simulink library "GFL_Lib"  (R2021a)
settings: Solver=VariableStepAuto  StartTime=0.0  StopTime=10.0  RelTol=1e-3
values from neighbouring files (symbols this model uses):
  Ki_i = Rc_eq*wn_i    [Init_GFL.m]
  Kp_i = Lc_eq/wb*wn_i    [Init_GFL.m]
  Lc_eq = Lc_pu + dLc_pu    [Init_VI_mmc.m]
  Lc_pu = Lt_pu+Larm_pu/2    [Init_VI_mmc.m]
  Lf_pu = Lc_eq    [Init_GFL.m]
  Va0 = sqrt(2)*Vb1*Vvsc0*sin(Theta_vsc0*pi/180)    [Init_LF_LCL_old.m]
  Vb0 = sqrt(2)*Vb1*Vvsc0*sin(Theta_vsc0*pi/180-2*pi/3)    [Init_LF_LCL_old.m]
  Vc0 = sqrt(2)*Vb1*Vvsc0*sin(Theta_vsc0*pi/180+2*pi/3)    [Init_LF_LCL_old.m]
  Vm0_d = Vvsc0 * cos(Theta_vsc0*pi/180-Theta_m0*pi/180)    [Init_LF_LCL_old.m]
  Vm0_q = Vvsc0 * sin(Theta_vsc0*pi/180-Theta_m0*pi/180)    [Init_LF_LCL_old.m]
  Vvsc0 = abs(Vm)    [Init_LF_LCL_old.m]
undefined symbols (not defined in the file or in its folder): Carm, Diff_CC_ki, Diff_CC_kp, fb, Ib2, Idcb, Ki_Wdiff_pu, Ki_Wtot_pu, Kp_Rvi_pu, Kp_Wdiff_pu, Kp_Wtot_pu, Lb, Sb, Solver_Time_Step, Time_Step, Vb1, Vb2, Vdcb, Vm0, VSC01_id0, wb, Zb
libraries: Control_Lib x57, spsVoltageMeasurementLib x17, spsSeriesRLCBranchLib x14, spsThreePhaseSourceLib x12, spsThreePhaseBreakerLib x10, spsThreePhaseVIMeasurementLib x9, spsThreePhaseTransformerTwoWindingsLib x7, spsCurrentMeasurementLib x7, powerlib x7, spsControlledCurrentSourceLib x6, spsControlledVoltageSourceLib x6, slpidlib x6
(part 5 of 6)

== system GFL_Lib/Mean Model 2-Level L-filter_old/Control loops/LPF3 ==
  In1 : Inport
  Add : Sum  Inputs=+-
  Gain : Gain  Gain=2*pi*50
  Integrator : Integrator  InitialCondition=V0
  Out1 : Outport
  wires:
  In1/1 -> Add/1
  Integrator/1 -> Add/2, Out1/1
  Gain/1 -> Integrator/1
  Add/1 -> Gain/1

== system GFL_Lib/Mean Model 2-Level L-filter_old/Control loops/RMS derivation ==
  dq : Inport
  Demux : Demux  Outputs=2
  Sqrt : Sqrt  SaturateOnIntegerOverflow=on
  Square : Math  Operator=square  SaturateOnIntegerOverflow=on
  Square1 : Math  Operator=square  SaturateOnIntegerOverflow=on
  Sum : Sum
  rms : Outport
  wires:
  dq/1 -> Demux/1
  Demux/2 -> Square1/1
  Square/1 -> Sum/1
  Demux/1 -> Square/1
  Sqrt/1 -> rms/1
  Sum/1 -> Sqrt/1
  Square1/1 -> Sum/2

== system GFL_Lib/Mean Model 2-Level L-filter_old/Control loops/norm1 ==
  In1 : Inport
  Add : Sum
  Demux : Demux  Outputs=2
  Sqrt : Sqrt  SaturateOnIntegerOverflow=on
  Square : Math  Operator=square  SaturateOnIntegerOverflow=on
  Square1 : Math  Operator=square  SaturateOnIntegerOverflow=on
  Out1 : Outport
  wires:
  In1/1 -> Demux/1
  Square1/1 -> Add/2
  Square/1 -> Add/1
  Demux/1 -> Square/1
  Demux/2 -> Square1/1
  Add/1 -> Sqrt/1
  Sqrt/1 -> Out1/1

== system GFL_Lib/Mean Model 2-Level L-filter_old/Control loops/norm2 ==
  In1 : Inport
  Add : Sum
  Demux : Demux  Outputs=2
  Sqrt : Sqrt  SaturateOnIntegerOverflow=on
  Square : Math  Operator=square  SaturateOnIntegerOverflow=on
  Square1 : Math  Operator=square  SaturateOnIntegerOverflow=on
  Out1 : Outport
  wires:
  In1/1 -> Demux/1
  Square1/1 -> Add/2
  Square/1 -> Add/1
  Demux/1 -> Square/1
  Demux/2 -> Square1/1
  Add/1 -> Sqrt/1
  Sqrt/1 -> Out1/1

== system GFL_Lib/Mean Model 2-Level L-filter_sav/Control loops/ pu P//Q computation ==
  v_abc_pu : Inport  PortDimensions=3
  i_abc_pu : Inport  Port=2  PortDimensions=3
  Demux : Demux  Outputs=3
      settings: DisplayOption=none
  Mux : Mux  Inputs=3
  Product1 : Product  InputSameDT=on  SaturateOnIntegerOverflow=on  OutDataTypeStr=Inherit: Same as first input
  Product3 : Product  InputSameDT=on  SaturateOnIntegerOverflow=on  OutDataTypeStr=Inherit: Same as first input
  Sum : Sum  Inputs=+-  InputSameDT=on  SaturateOnIntegerOverflow=on  OutDataTypeStr=Inherit: Same as first input
  Sum1 : Sum  Inputs=1  InputSameDT=on  SaturateOnIntegerOverflow=on  OutDataTypeStr=Inherit: Same as first input
  Sum4 : Sum  Inputs=1  InputSameDT=on  SaturateOnIntegerOverflow=on  OutDataTypeStr=Inherit: Same as first input
  Sum5 : Sum  Inputs=+-  InputSameDT=on  SaturateOnIntegerOverflow=on  OutDataTypeStr=Inherit: Same as first input
  Sum6 : Sum  Inputs=+-  InputSameDT=on  SaturateOnIntegerOverflow=on  OutDataTypeStr=Inherit: Same as first input
  pu->V : Gain  Gain=1/sqrt(3)  SaturateOnIntegerOverflow=on  OutDataTypeStr=Inherit: Same as input  ParamDataTypeStr=Inherit: Same as input
  pu->V1 : Gain  Gain=1/3  SaturateOnIntegerOverflow=on  OutDataTypeStr=Inherit: Same as input  ParamDataTypeStr=Inherit: Same as input
  pu->V2 : Gain  Gain=1/3  SaturateOnIntegerOverflow=on  OutDataTypeStr=Inherit: Same as input  ParamDataTypeStr=Inherit: Same as input
  P : Outport  VectorParamsAs1DForOutWhenUnconnected=off
  Q : Outport  Port=2  VectorParamsAs1DForOutWhenUnconnected=off
  wires:
  pu->V2/1 -> Q/1
  pu->V1/1 -> P/1
  Sum1/1 -> pu->V/1
  Product3/1 -> Sum1/1
  Product1/1 -> Sum4/1
  v_abc_pu/1 -> Product1/1, Demux/1
  i_abc_pu/1 -> Product1/2, Product3/2
  Sum4/1 -> pu->V1/1
  Demux/1 -> Sum/1, Sum6/2
  Demux/2 -> Sum/2, Sum5/1
  Demux/3 -> Sum5/2, Sum6/1
  Sum/1 -> Mux/3
  Sum5/1 -> Mux/1
  Sum6/1 -> Mux/2
  Mux/1 -> Product3/1
  pu->V/1 -> pu->V2/1  "Q"

== system GFL_Lib/Mean Model 2-Level L-filter_sav/Control loops/Inner Current Control ==
  ig_dq_ref : Inport
  ig_dq : Inport  Port=2
  theta_PLL : Inport  Port=3
  w_PLL : Inport  Port=4
  vg_dq : Inport  Port=5
  Control Delay compensation : Constant  Value=wb*Solver_Time_Step
  Current PI control : Subsystem
  Mux : Mux  Inputs=2
  Sum : Sum  Inputs=|++
  Trigonometric Function : Trigonometry
  Trigonometric Function1 : Trigonometry  Operator=cos
  vm_dq : Outport  VectorParamsAs1DForOutWhenUnconnected=off
  CosSinTheta_delay : Outport  Port=2  VectorParamsAs1DForOutWhenUnconnected=off
  wires:
  ig_dq/1 -> Current PI control/1(Is_dq)  "Is_dq"
  Current PI control/1(vm_dq_ref) -> vm_dq/1  "vm_dq"
  ig_dq_ref/1 -> Current PI control/3(Is_dq_ref)
  vg_dq/1 -> Current PI control/2(Eg_dqfr)  "Eg_dq"
  w_PLL/1 -> Current PI control/4(w)  "w"
  Control Delay compensation/1 -> Sum/2
  Trigonometric Function/1 -> Mux/2
  Sum/1 -> Trigonometric Function/1, Trigonometric Function1/1
  theta_PLL/1 -> Sum/1  "Theta"
  Trigonometric Function1/1 -> Mux/1
  Mux/1 -> CosSinTheta_delay/1

== system GFL_Lib/Mean Model 2-Level LCL-filter [under construction]/Control loops/ pu P//Q computation ==
  v_abc_pu : Inport  PortDimensions=3
  i_abc_pu : Inport  Port=2  PortDimensions=3
  Demux : Demux  Outputs=3
      settings: DisplayOption=none
  Mux : Mux  Inputs=3
  Product1 : Product  InputSameDT=on  SaturateOnIntegerOverflow=on  OutDataTypeStr=Inherit: Same as first input
  Product3 : Product  InputSameDT=on  SaturateOnIntegerOverflow=on  OutDataTypeStr=Inherit: Same as first input
  Sum : Sum  Inputs=+-  InputSameDT=on  SaturateOnIntegerOverflow=on  OutDataTypeStr=Inherit: Same as first input
  Sum1 : Sum  Inputs=1  InputSameDT=on  SaturateOnIntegerOverflow=on  OutDataTypeStr=Inherit: Same as first input
  Sum4 : Sum  Inputs=1  InputSameDT=on  SaturateOnIntegerOverflow=on  OutDataTypeStr=Inherit: Same as first input
  Sum5 : Sum  Inputs=+-  InputSameDT=on  SaturateOnIntegerOverflow=on  OutDataTypeStr=Inherit: Same as first input
  Sum6 : Sum  Inputs=+-  InputSameDT=on  SaturateOnIntegerOverflow=on  OutDataTypeStr=Inherit: Same as first input
  pu->V : Gain  Gain=1/sqrt(3)  SaturateOnIntegerOverflow=on  OutDataTypeStr=Inherit: Same as input  ParamDataTypeStr=Inherit: Same as input
  pu->V1 : Gain  Gain=1/3  SaturateOnIntegerOverflow=on  OutDataTypeStr=Inherit: Same as input  ParamDataTypeStr=Inherit: Same as input
  pu->V2 : Gain  Gain=1/3  SaturateOnIntegerOverflow=on  OutDataTypeStr=Inherit: Same as input  ParamDataTypeStr=Inherit: Same as input
  P : Outport  VectorParamsAs1DForOutWhenUnconnected=off
  Q : Outport  Port=2  VectorParamsAs1DForOutWhenUnconnected=off
  wires:
  pu->V2/1 -> Q/1
  pu->V1/1 -> P/1
  Sum1/1 -> pu->V/1
  Product3/1 -> Sum1/1
  Product1/1 -> Sum4/1
  v_abc_pu/1 -> Product1/1, Demux/1
  i_abc_pu/1 -> Product1/2, Product3/2
  Sum4/1 -> pu->V1/1
  Demux/1 -> Sum/1, Sum6/2
  Demux/2 -> Sum/2, Sum5/1
  Demux/3 -> Sum5/2, Sum6/1
  Sum/1 -> Mux/3
  Sum5/1 -> Mux/1
  Sum6/1 -> Mux/2
  Mux/1 -> Product3/1
  pu->V/1 -> pu->V2/1  "Q"

== system GFL_Lib/Mean Model 2-Level LCL-filter [under construction]/Control loops/Inner Current Control ==
  ig_dq_ref : Inport
  ig_dq : Inport  Port=2
  theta_PLL : Inport  Port=3
  w_PLL : Inport  Port=4
  vg_dq : Inport  Port=5
  Current PI control : Subsystem
  vm_dq : Outport  VectorParamsAs1DForOutWhenUnconnected=off
  theta : Outport  Port=2  VectorParamsAs1DForOutWhenUnconnected=off
  wires:
  ig_dq/1 -> Current PI control/1(Is_dq)  "Is_dq"
  theta_PLL/1 -> theta/1  "Theta"
  Current PI control/1(vm_dq_ref) -> vm_dq/1  "vm_dq"
  ig_dq_ref/1 -> Current PI control/3(Is_dq_ref)
  vg_dq/1 -> Current PI control/2(Eg_dqfr)  "Eg_dq"
  w_PLL/1 -> Current PI control/4(w)  "w"

== system GFL_Lib/GFL IDEAL VSC/Control loops/Inner Current Control/LPF1 ==
  In1 : Inport
  Add : Sum  Inputs=+-
  Gain : Gain  Gain=w_ff
  Integrator : Integrator  InitialConditionSource=external  InitialCondition=V0*cos(Theta0*pi/180)
  Out1 : Outport
  wires:
  Add/1 -> Gain/1
  Gain/1 -> Integrator/1
  Integrator/1 -> Out1/1, Add/2
  In1/1 -> Integrator/2, Add/1

== system GFL_Lib/GFL IDEAL VSC/Control loops/Inner Current Control/LPF2 ==
  In1 : Inport
  Add : Sum  Inputs=+-
  Gain : Gain  Gain=w_ff
  Integrator : Integrator  InitialCondition=V0*sin(Theta0*pi/180)
  Out1 : Outport
  wires:
  Add/1 -> Gain/1
  Gain/1 -> Integrator/1
  Integrator/1 -> Out1/1, Add/2
  In1/1 -> Add/1

== system GFL_Lib/GFL MMC/Control loops/Inner Current Control/LPF1 ==
  In1 : Inport
  Add : Sum  Inputs=+-
  Gain : Gain  Gain=w_ff
  Integrator : Integrator  InitialConditionSource=external  InitialCondition=V0*cos(Theta0*pi/180)
  Out1 : Outport
  wires:
  Add/1 -> Gain/1
  Gain/1 -> Integrator/1
  Integrator/1 -> Out1/1, Add/2
  In1/1 -> Integrator/2, Add/1

== system GFL_Lib/GFL MMC/Control loops/Inner Current Control/LPF2 ==
  In1 : Inport
  Add : Sum  Inputs=+-
  Gain : Gain  Gain=w_ff
  Integrator : Integrator  InitialCondition=V0*sin(Theta0*pi/180)
  Out1 : Outport
  wires:
  Add/1 -> Gain/1
  Gain/1 -> Integrator/1
  Integrator/1 -> Out1/1, Add/2
  In1/1 -> Add/1

== system GFL_Lib/GFM_VC MMC/Bridge_Model/MMC Average Model/Arm_la ==
  m : Inport
  Controlled Current Source : spsControlledCurrentSourceLib/Controlled Current Source  Initialize=on  Source_Type=DC  Amplitude=0  Phase=0  Frequency=0  Measurements=None
  Controlled Voltage Source2 : spsControlledVoltageSourceLib/Controlled Voltage Source  Initialize=on  Source_Type=DC  Amplitude=Vdc/2  Phase=180  Frequency=0  Measurements=None
  Current Measurement7 : spsCurrentMeasurementLib/Current Measurement  PhasorSimulation=off  OutputType=Complex  PSBequivalent=0
  Memory1 : Memory  InitialCondition=Vdc/2
  Memory2 : Memory
  Product : Product  RndMeth=Zero
  Product1 : Product  RndMeth=Zero
  Series RLC Branch : spsSeriesRLCBranchLib/Series RLC Branch  LConnTagsString=__new0  RConnTagsString=__new0  BranchType=C  Resistance=1  Inductance=1e-3  SetiL0=off  InitialCurrent=0  Capacitance=C_arm  Setx0=on  InitialVoltage=Vdc  Measurements=None
  Voltage Measurement : spsVoltageMeasurementLib/Voltage Measurement  PhasorSimulation=off  OutputType=Complex  PSBequivalent=0
  Voltage Measurement1 : spsVoltageMeasurementLib/Voltage Measurement  PhasorSimulation=off  OutputType=Complex  PSBequivalent=0
  V+ : PMIOPort  Side=Left
  V- : PMIOPort  Port=2  Side=Left
  vctot : Outport
  i_arm : Outport  Port=2
  v_arm : Outport  Port=3
  wires:
  Memory1/1 -> Controlled Voltage Source2/1
  Memory2/1 -> Controlled Current Source/1
  Product/1 -> Memory1/1
  Voltage Measurement/1 -> v_arm/1
  Product1/1 -> Memory2/1
  m/1 -> [m], Product1/1
  Current Measurement7/1 -> i_arm/1, Product1/2
  [m] -> Product/2
  Voltage Measurement1/1 -> Product/1, vctot/1
  connections:
  Current Measurement7/RConn1 -- Controlled Voltage Source2/RConn1
  Current Measurement7/LConn1 -- Voltage Measurement/LConn1 -- V+/RConn1
  Controlled Current Source/LConn1 -- Series RLC Branch/RConn1 -- Voltage Measurement1/LConn2 -- V-/RConn1 -- Voltage Measurement/LConn2 -- Controlled Voltage Source2/LConn1
  Controlled Current Source/RConn1 -- Series RLC Branch/LConn1 -- Voltage Measurement1/LConn1

== system GFL_Lib/GFM_VC MMC/Bridge_Model/MMC Average Model/Arm_lb ==
  m : Inport
  Controlled Current Source : spsControlledCurrentSourceLib/Controlled Current Source  Initialize=on  Source_Type=DC  Amplitude=0  Phase=0  Frequency=0  Measurements=None
  Controlled Voltage Source2 : spsControlledVoltageSourceLib/Controlled Voltage Source  Initialize=on  Source_Type=DC  Amplitude=Vdc/2  Phase=180  Frequency=0  Measurements=None
  Current Measurement7 : spsCurrentMeasurementLib/Current Measurement  PhasorSimulation=off  OutputType=Complex  PSBequivalent=0
  Memory1 : Memory  InitialCondition=Vdc/2
  Memory2 : Memory
  Product : Product  RndMeth=Zero
  Product1 : Product  RndMeth=Zero
  Series RLC Branch : spsSeriesRLCBranchLib/Series RLC Branch  LConnTagsString=__new0  RConnTagsString=__new0  BranchType=C  Resistance=1  Inductance=1e-3  SetiL0=off  InitialCurrent=0  Capacitance=C_arm  Setx0=on  InitialVoltage=Vdc  Measurements=None
  Voltage Measurement : spsVoltageMeasurementLib/Voltage Measurement  PhasorSimulation=off  OutputType=Complex  PSBequivalent=0
  Voltage Measurement1 : spsVoltageMeasurementLib/Voltage Measurement  PhasorSimulation=off  OutputType=Complex  PSBequivalent=0
  V+ : PMIOPort  Side=Left
  V- : PMIOPort  Port=2  Side=Left
  vctot : Outport
  i_arm : Outport  Port=2
  v_arm : Outport  Port=3
  wires:
  Memory1/1 -> Controlled Voltage Source2/1
  Memory2/1 -> Controlled Current Source/1
  Product/1 -> Memory1/1
  Voltage Measurement/1 -> v_arm/1
  Product1/1 -> Memory2/1
  m/1 -> [m], Product1/1
  Current Measurement7/1 -> i_arm/1, Product1/2
  [m] -> Product/2
  Voltage Measurement1/1 -> Product/1, vctot/1
  connections:
  Current Measurement7/RConn1 -- Controlled Voltage Source2/RConn1
  Current Measurement7/LConn1 -- Voltage Measurement/LConn1 -- V+/RConn1
  Controlled Current Source/LConn1 -- Series RLC Branch/RConn1 -- Voltage Measurement1/LConn2 -- V-/RConn1 -- Voltage Measurement/LConn2 -- Controlled Voltage Source2/LConn1
  Controlled Current Source/RConn1 -- Series RLC Branch/LConn1 -- Voltage Measurement1/LConn1

== system GFL_Lib/GFM_VC MMC/Bridge_Model/MMC Average Model/Arm_lc ==
  m : Inport
  Controlled Current Source : spsControlledCurrentSourceLib/Controlled Current Source  Initialize=on  Source_Type=DC  Amplitude=0  Phase=0  Frequency=0  Measurements=None
  Controlled Voltage Source2 : spsControlledVoltageSourceLib/Controlled Voltage Source  Initialize=on  Source_Type=DC  Amplitude=Vdc/2  Phase=180  Frequency=0  Measurements=None
  Current Measurement7 : spsCurrentMeasurementLib/Current Measurement  PhasorSimulation=off  OutputType=Complex  PSBequivalent=0
  Memory1 : Memory  InitialCondition=Vdc/2
  Memory2 : Memory
  Product : Product  RndMeth=Zero
  Product1 : Product  RndMeth=Zero
  Series RLC Branch : spsSeriesRLCBranchLib/Series RLC Branch  LConnTagsString=__new0  RConnTagsString=__new0  BranchType=C  Resistance=1  Inductance=1e-3  SetiL0=off  InitialCurrent=0  Capacitance=C_arm  Setx0=on  InitialVoltage=Vdc  Measurements=None
  Voltage Measurement : spsVoltageMeasurementLib/Voltage Measurement  PhasorSimulation=off  OutputType=Complex  PSBequivalent=0
  Voltage Measurement1 : spsVoltageMeasurementLib/Voltage Measurement  PhasorSimulation=off  OutputType=Complex  PSBequivalent=0
  V+ : PMIOPort  Side=Left
  V- : PMIOPort  Port=2  Side=Left
  vctot : Outport
  i_arm : Outport  Port=2
  v_arm : Outport  Port=3
  wires:
  Memory1/1 -> Controlled Voltage Source2/1
  Memory2/1 -> Controlled Current Source/1
  Product/1 -> Memory1/1
  Voltage Measurement/1 -> v_arm/1
  Product1/1 -> Memory2/1
  m/1 -> [m], Product1/1
  Current Measurement7/1 -> i_arm/1, Product1/2
  [m] -> Product/2
  Voltage Measurement1/1 -> Product/1, vctot/1
  connections:
  Current Measurement7/RConn1 -- Controlled Voltage Source2/RConn1
  Current Measurement7/LConn1 -- Voltage Measurement/LConn1 -- V+/RConn1
  Controlled Current Source/LConn1 -- Series RLC Branch/RConn1 -- Voltage Measurement1/LConn2 -- V-/RConn1 -- Voltage Measurement/LConn2 -- Controlled Voltage Source2/LConn1
  Controlled Current Source/RConn1 -- Series RLC Branch/LConn1 -- Voltage Measurement1/LConn1

== system GFL_Lib/GFM_VC MMC/Bridge_Model/MMC Average Model/Arm_ua ==
  m : Inport
  Controlled Current Source : spsControlledCurrentSourceLib/Controlled Current Source  Initialize=on  Source_Type=DC  Amplitude=0  Phase=0  Frequency=0  Measurements=None
  Controlled Voltage Source2 : spsControlledVoltageSourceLib/Controlled Voltage Source  Initialize=on  Source_Type=DC  Amplitude=Vdc/2  Phase=180  Frequency=0  Measurements=None
  Current Measurement7 : spsCurrentMeasurementLib/Current Measurement  PhasorSimulation=off  OutputType=Complex  PSBequivalent=0
  Memory1 : Memory  InitialCondition=Vdc/2
  Memory2 : Memory
  Product : Product  RndMeth=Zero
  Product1 : Product  RndMeth=Zero
  Series RLC Branch : spsSeriesRLCBranchLib/Series RLC Branch  LConnTagsString=__new0  RConnTagsString=__new0  BranchType=C  Resistance=1  Inductance=1e-3  SetiL0=off  InitialCurrent=0  Capacitance=C_arm  Setx0=on  InitialVoltage=Vdc  Measurements=None
  Voltage Measurement : spsVoltageMeasurementLib/Voltage Measurement  PhasorSimulation=off  OutputType=Complex  PSBequivalent=0
  Voltage Measurement1 : spsVoltageMeasurementLib/Voltage Measurement  PhasorSimulation=off  OutputType=Complex  PSBequivalent=0
  V+ : PMIOPort  Side=Left
  V- : PMIOPort  Port=2  Side=Left
  vctot : Outport
  i_arm : Outport  Port=2
  v_arm : Outport  Port=3
  wires:
  Memory1/1 -> Controlled Voltage Source2/1
  Memory2/1 -> Controlled Current Source/1
  Product/1 -> Memory1/1
  Voltage Measurement/1 -> v_arm/1
  Product1/1 -> Memory2/1
  m/1 -> [m], Product1/1
  Current Measurement7/1 -> i_arm/1, Product1/2
  [m] -> Product/2
  Voltage Measurement1/1 -> Product/1, vctot/1
  connections:
  Current Measurement7/RConn1 -- Controlled Voltage Source2/RConn1
  Current Measurement7/LConn1 -- Voltage Measurement/LConn1 -- V+/RConn1
  Controlled Current Source/LConn1 -- Series RLC Branch/RConn1 -- Voltage Measurement1/LConn2 -- V-/RConn1 -- Voltage Measurement/LConn2 -- Controlled Voltage Source2/LConn1
  Controlled Current Source/RConn1 -- Series RLC Branch/LConn1 -- Voltage Measurement1/LConn1

== system GFL_Lib/GFM_VC MMC/Bridge_Model/MMC Average Model/Arm_ub ==
  m : Inport
  Controlled Current Source : spsControlledCurrentSourceLib/Controlled Current Source  Initialize=on  Source_Type=DC  Amplitude=0  Phase=0  Frequency=0  Measurements=None
  Controlled Voltage Source2 : spsControlledVoltageSourceLib/Controlled Voltage Source  Initialize=on  Source_Type=DC  Amplitude=Vdc/2  Phase=180  Frequency=0  Measurements=None
  Current Measurement7 : spsCurrentMeasurementLib/Current Measurement  PhasorSimulation=off  OutputType=Complex  PSBequivalent=0
  Memory1 : Memory  InitialCondition=Vdc/2
  Memory2 : Memory
  Product : Product  RndMeth=Zero
  Product1 : Product  RndMeth=Zero
  Series RLC Branch : spsSeriesRLCBranchLib/Series RLC Branch  LConnTagsString=__new0  RConnTagsString=__new0  BranchType=C  Resistance=1  Inductance=1e-3  SetiL0=off  InitialCurrent=0  Capacitance=C_arm  Setx0=on  InitialVoltage=Vdc  Measurements=None
  Voltage Measurement : spsVoltageMeasurementLib/Voltage Measurement  PhasorSimulation=off  OutputType=Complex  PSBequivalent=0
  Voltage Measurement1 : spsVoltageMeasurementLib/Voltage Measurement  PhasorSimulation=off  OutputType=Complex  PSBequivalent=0
  V+ : PMIOPort  Side=Left
  V- : PMIOPort  Port=2  Side=Left
  vctot : Outport
  i_arm : Outport  Port=2
  v_arm : Outport  Port=3
  wires:
  Memory1/1 -> Controlled Voltage Source2/1
  Memory2/1 -> Controlled Current Source/1
  Product/1 -> Memory1/1
  Voltage Measurement/1 -> v_arm/1
  Product1/1 -> Memory2/1
  m/1 -> [m], Product1/1
  Current Measurement7/1 -> i_arm/1, Product1/2
  [m] -> Product/2
  Voltage Measurement1/1 -> Product/1, vctot/1
  connections:
  Current Measurement7/RConn1 -- Controlled Voltage Source2/RConn1
  Current Measurement7/LConn1 -- Voltage Measurement/LConn1 -- V+/RConn1
  Controlled Current Source/LConn1 -- Series RLC Branch/RConn1 -- Voltage Measurement1/LConn2 -- V-/RConn1 -- Voltage Measurement/LConn2 -- Controlled Voltage Source2/LConn1
  Controlled Current Source/RConn1 -- Series RLC Branch/LConn1 -- Voltage Measurement1/LConn1

== system GFL_Lib/GFM_VC MMC/Bridge_Model/MMC Average Model/Arm_uc ==
  m : Inport
  Controlled Current Source : spsControlledCurrentSourceLib/Controlled Current Source  Initialize=on  Source_Type=DC  Amplitude=0  Phase=0  Frequency=0  Measurements=None
  Controlled Voltage Source2 : spsControlledVoltageSourceLib/Controlled Voltage Source  Initialize=on  Source_Type=DC  Amplitude=Vdc/2  Phase=180  Frequency=0  Measurements=None
  Current Measurement7 : spsCurrentMeasurementLib/Current Measurement  PhasorSimulation=off  OutputType=Complex  PSBequivalent=0
  Memory1 : Memory  InitialCondition=Vdc/2
  Memory2 : Memory
  Product : Product  RndMeth=Zero
  Product1 : Product  RndMeth=Zero
  Series RLC Branch : spsSeriesRLCBranchLib/Series RLC Branch  LConnTagsString=__new0  RConnTagsString=__new0  BranchType=C  Resistance=1  Inductance=1e-3  SetiL0=off  InitialCurrent=0  Capacitance=C_arm  Setx0=on  InitialVoltage=Vdc  Measurements=None
  Voltage Measurement : spsVoltageMeasurementLib/Voltage Measurement  PhasorSimulation=off  OutputType=Complex  PSBequivalent=0
  Voltage Measurement1 : spsVoltageMeasurementLib/Voltage Measurement  PhasorSimulation=off  OutputType=Complex  PSBequivalent=0
  V+ : PMIOPort  Side=Left
  V- : PMIOPort  Port=2  Side=Left
  vctot : Outport
  i_arm : Outport  Port=2
  v_arm : Outport  Port=3
  wires:
  Memory1/1 -> Controlled Voltage Source2/1
  Memory2/1 -> Controlled Current Source/1
  Product/1 -> Memory1/1
  Voltage Measurement/1 -> v_arm/1
  Product1/1 -> Memory2/1
  m/1 -> [m], Product1/1
  Current Measurement7/1 -> i_arm/1, Product1/2
  [m] -> Product/2
  Voltage Measurement1/1 -> Product/1, vctot/1
  connections:
  Current Measurement7/RConn1 -- Controlled Voltage Source2/RConn1
  Current Measurement7/LConn1 -- Voltage Measurement/LConn1 -- V+/RConn1
  Controlled Current Source/LConn1 -- Series RLC Branch/RConn1 -- Voltage Measurement1/LConn2 -- V-/RConn1 -- Voltage Measurement/LConn2 -- Controlled Voltage Source2/LConn1
  Controlled Current Source/RConn1 -- Series RLC Branch/LConn1 -- Voltage Measurement1/LConn1

== system GFL_Lib/GFM_VC MMC/Control loops/Current Limitation/Current control ==
  Ig_dq0* : Inport
  Ig_dq0 : Inport  Port=2
  vg_dq0 : Inport  Port=3
  w : Inport  Port=4
  Demux : Demux  Outputs=2
  Demux1 : Demux  Outputs=2
  Demux2 : Demux  Outputs=2
  Gain Corrector : Gain  Gain=3/(Tr_I_max/1000)*(Lt_pu+Larm_pu/2)/wb
  Gain Corrector1 : Gain  Gain=3/(Tr_I_max/1000)*(Lt_pu+Larm_pu/2)/wb
  Mux : Mux  Inputs=2
  Product : Product  RndMeth=Zero
  Product1 : Product  RndMeth=Zero
  Sum : Sum  Inputs=|+-
  Sum2 : Sum  Inputs=|+-
  Sum3 : Sum  Inputs=|++
  Sum5 : Sum  Inputs=++|
  Sum6 : Sum  Inputs=-+|
  Sum7 : Sum  Inputs=++|
  vpcc_abc{1,3..6} (5 alike) : Scope
  w*Lf_pu : Gain  Gain=Lt_pu
  vm : Outport  InitialOutput=0  VectorParamsAs1DForOutWhenUnconnected=off
  wires:
  Demux2/2 -> Sum7/1
  Demux2/1 -> Sum3/2
  w/1 -> vpcc_abc5/1, w*Lf_pu/1
  Sum/1 -> vpcc_abc1/1, Gain Corrector/1
  Sum7/1 -> Mux/2  "Vm_q*"
  Sum3/1 -> Mux/1, vpcc_abc3/1  "Vm_d*"
  Sum5/1 -> Sum7/2
  Product1/1 -> Sum5/1
  Gain Corrector1/1 -> Sum5/2
  Demux/2 -> Sum6/2
  Sum2/1 -> Sum3/1
  Product/1 -> Sum2/2
  Demux1/2 -> Sum6/1, Product/1
  w*Lf_pu/1 -> Product/2, Product1/1
  Gain Corrector/1 -> Sum2/1
  Demux1/1 -> Sum/2, Product1/2
  Demux/1 -> Sum/1
  Ig_dq0/1 -> Demux1/1
  vg_dq0/1 -> Demux2/1, vpcc_abc6/1
  Sum6/1 -> Gain Corrector1/1
  Ig_dq0*/1 -> vpcc_abc4/1, Demux/1
  Mux/1 -> vm/1

== system GFL_Lib/GFM_VC MMC/Control loops/Current Limitation/Inverse Current control ==
  Vm_dq* : Inport
  Ig_dq : Inport  Port=2
  vg_dq : Inport  Port=3
  w : Inport  Port=4
  Demux : Demux  Outputs=2
  Demux1 : Demux  Outputs=2
  Demux2 : Demux  Outputs=2
  Gain Corrector2 : Gain  Gain=1/(3/(Tr_I_max/1000)*(Lt_pu+Larm_pu/2)/wb)
  Gain Corrector3 : Gain  Gain=1/(3/(Tr_I_max/1000)*(Lt_pu+Larm_pu/2)/wb)
  Mux : Mux  Inputs=2
  Product : Product  RndMeth=Zero
  Product1 : Product  RndMeth=Zero
  Sum : Sum  Inputs=|+-
  Sum2 : Sum  Inputs=|++
  Sum3 : Sum  Inputs=|++
  Sum5 : Sum  Inputs=-+|
  Sum6 : Sum  Inputs=-+|
  Sum7 : Sum  Inputs=++|
  w*Lf_pu : Gain  Gain=Lt_pu
  Is_dq* : Outport  InitialOutput=0  VectorParamsAs1DForOutWhenUnconnected=off
  wires:
  vg_dq/1 -> Demux2/1
  Ig_dq/1 -> Demux1/1
  Vm_dq*/1 -> Demux/1
  Demux/1 -> Sum/1
  Demux1/1 -> Sum3/2, Product1/2
  Sum/1 -> Sum2/1
  w*Lf_pu/1 -> Product1/1, Product/2
  Product/1 -> Sum2/2
  Sum2/1 -> Gain Corrector3/1
  Mux/1 -> Is_dq*/1
  Demux/2 -> Sum6/2
  Sum6/1 -> Sum5/2
  Sum5/1 -> Gain Corrector2/1
  Sum3/1 -> Mux/1  "is_d*"
  Sum7/1 -> Mux/2  "is_q*"
  w/1 -> w*Lf_pu/1
  Demux1/2 -> Sum7/1, Product/1
  Gain Corrector3/1 -> Sum3/1
  Demux2/1 -> Sum/2
  Demux2/2 -> Sum6/1
  Product1/1 -> Sum5/1
  Gain Corrector2/1 -> Sum7/2

== system GFL_Lib/GFM_VC MMC/Control loops/DC part: stored energy control + differential current control/Control Wdiff ==
  note: Matrix transformation
      | to cancel homopolar
  Wdiff pu : Inport
  Wdiff_ref pu : Inport  Port=2
  theta : Inport  Port=3
  Gain : Gain  Gain=-1
  Gain2 : Gain  Gain=-2
  Gain_i 1 : Gain  Gain=Ki_Wdiff_pu  SaturateOnIntegerOverflow=on  OutDataTypeStr=Inherit: Same as input  ParamDataTypeStr=Inherit: Same as input
  Gain_i 4 : Gain  Gain=Kp_Wdiff_pu  SaturateOnIntegerOverflow=on  OutDataTypeStr=Inherit: Same as input  ParamDataTypeStr=Inherit: Same as input
  Integrator : Integrator  InitialConditionSource=external
  Mux1 : Mux  Inputs=3
  Mux2 : Mux  Inputs=3
  Mux3 : Mux  Commented=on  Inputs=3
  Mux5 : Mux  Inputs=2
  Sum2 : Sum  InputSameDT=on  SaturateOnIntegerOverflow=on  OutDataTypeStr=Inherit: Same as first input
  Sum3 : Sum  Inputs=+-  InputSameDT=on  SaturateOnIntegerOverflow=on  OutDataTypeStr=Inherit: Same as first input
  vsa_1 : Fcn  Expr=u(1)*sin(u(4))
  vsa_2 : Fcn  Expr=u(1)-1/2*u(2)-1/2*u(3)
  vsa_3 : Fcn  Commented=on  Expr=u(1)*cos(u(4))+1/3^0.5*u(2)*cos(u(4)+1/2*pi)+1/3^0.5*u(3)*cos(u(4)-1/2*pi)
  vsb_1 : Fcn  Expr=-1/2*u(1)+u(2)-1/2*u(3)
  vsb_2 : Fcn  Expr=u(2)*sin(u(4)-2/3*pi)
  vsb_3 : Fcn  Expr=u(3)*sin(u(4)+2/3*pi)
  vsb_4 : Fcn  Expr=-1/2*u(1)-1/2*u(2)+u(3)
  vsb_5 : Fcn  Commented=on  Expr=1/3^0.5*u(1)*cos(u(4)-7/6*pi)+u(2)*cos(u(4)-2/3*pi)+1/3^0.5*u(3)*cos(u(4)-1/6*pi)
  vsb_6 : Fcn  Commented=on  Expr=1/3^0.5*u(1)*cos(u(4)+7/6*pi)+1/3^0.5*u(2)*cos(u(4)+1/6*pi)+u(3)*cos(u(4)+2/3*pi)
  Idiff ref pu : Outport
  wires:
  Mux2/1 -> Idiff ref pu/1
  Gain/1 -> Integrator/2
  Sum2/1 -> Gain2/1
  Wdiff pu/1 -> Sum3/2
  Wdiff_ref pu/1 -> Sum3/1
  vsb_2/1 -> Mux1/2
  vsa_1/1 -> Mux1/1
  vsb_3/1 -> Mux1/3
  Gain2/1 -> Mux5/1  "Idiff_ac_pu"
  vsa_2/1 -> Mux2/1
  vsb_1/1 -> Mux2/2
  vsb_4/1 -> Mux2/3
  vsb_6/1 -> Mux3/3
  vsa_3/1 -> Mux3/1
  vsb_5/1 -> Mux3/2
  Mux5/1 -> vsa_3/1, vsb_5/1, vsb_6/1, vsa_1/1, vsb_2/1, vsb_3/1
  theta/1 -> Mux5/2
  Integrator/1 -> Sum2/1
  Gain_i 1/1 -> Integrator/1
  Sum3/1 -> Gain_i 4/1, Gain_i 1/1
  Gain_i 4/1 -> Gain/1, Sum2/2
  Mux1/1 -> vsa_2/1, vsb_4/1, vsb_1/1

== system GFL_Lib/GFM_VC MMC/Control loops/DC part: stored energy control + differential current control/Control Wtot  ==
  note: Reference of i_diff --> adjusting dc power
  note: Energy based control
      |
      | dW
      | ----- = Pdc - Pac --> In this simulation, the energy is regulated by adjusting dc power
      | dt
      |
      | Pdc = PIcontroller*(W_ref - W_mes) + Pac
  note: ac power is considered as a disturbance
  Wtot_pu : Inport
  Wtot ref pu : Inport  Port=2
  p_ac_pu : Inport  Port=3
  Vdc_pu : Inport  Port=4
  Divide1 : Product  Inputs=/*
  Gain : Gain  Gain=-1
  Gain1 : Gain  Gain=1/3
  Gain_i 1 : Gain  Gain=Kp_Wtot_pu  SaturateOnIntegerOverflow=on  OutDataTypeStr=Inherit: Same as input  ParamDataTypeStr=Inherit: Same as input
  Gain_i 5 : Gain  Gain=Ki_Wtot_pu  SaturateOnIntegerOverflow=on  OutDataTypeStr=Inherit: Same as input  ParamDataTypeStr=Inherit: Same as input
  Integrator : Integrator  InitialConditionSource=external
  Sum : Sum  Inputs=++|
  Sum1 : Sum  InputSameDT=on  SaturateOnIntegerOverflow=on  OutDataTypeStr=Inherit: Same as first input
  Sum4 : Sum  Inputs=+-  InputSameDT=on  SaturateOnIntegerOverflow=on  OutDataTypeStr=Inherit: Same as first input
  Idiff ref pu : Outport
  wires:
  Gain/1 -> Integrator/2
  Sum/1 -> Divide1/2
  Divide1/1 -> Idiff ref pu/1  "idiff_ref"
  Vdc_pu/1 -> Divide1/1
  Sum1/1 -> Sum/2
  Sum4/1 -> Gain_i 1/1, Gain_i 5/1
  Gain_i 5/1 -> Integrator/1
  Integrator/1 -> Sum1/1
  Gain_i 1/1 -> Sum1/2, Gain/1
  Wtot ref pu/1 -> Sum4/1
  Wtot_pu/1 -> Sum4/2
  p_ac_pu/1 -> Gain1/1
  Gain1/1 -> Sum/1

== system GFL_Lib/GFM_VC MMC/Control loops/DC part: stored energy control + differential current control/Differential_current_control ==
  vdc_pu : Inport
  idiff_pu : Inport  Port=2
  idiff_ref_pu : Inport  Port=3
  Constant : Constant
  Gain3 : Gain  Gain=1/2
  Gain_i 1 : Gain  Gain=Diff_CC_kp  SaturateOnIntegerOverflow=on  OutDataTypeStr=Inherit: Same as input  ParamDataTypeStr=Inherit: Same as input
  Gain_i 5 : Gain  Gain=Diff_CC_ki  SaturateOnIntegerOverflow=on  OutDataTypeStr=Inherit: Same as input  ParamDataTypeStr=Inherit: Same as input
  Integrator : Integrator
  Scope : Scope  NumInputPorts=2
  Sum1 : Sum  Inputs=+-  InputSameDT=on  SaturateOnIntegerOverflow=on  OutDataTypeStr=Inherit: Same as first input
  Sum2 : Sum  InputSameDT=on  SaturateOnIntegerOverflow=on  OutDataTypeStr=Inherit: Same as first input
  Sum3 : Sum  Inputs=+-  InputSameDT=on  SaturateOnIntegerOverflow=on  OutDataTypeStr=Inherit: Same as first input
  Vprediff_ref_pu : Outport
  wires:
  idiff_pu/1 -> Sum1/2, Scope/2
  idiff_ref_pu/1 -> Sum1/1, Scope/1
  Sum1/1 -> Gain_i 1/1, Gain_i 5/1
  Gain_i 5/1 -> Integrator/1
  Gain_i 1/1 -> Sum2/2
  Integrator/1 -> Sum2/1
  Constant/1 -> Gain3/1
  Gain3/1 -> Sum3/1
  Sum3/1 -> Vprediff_ref_pu/1
  Sum2/1 -> Sum3/2

== system GFL_Lib/GFM_VC MMC/Control loops/DC part: stored energy control + differential current control/Wdiff computation ==
  vctot u_pu : Inport
  vctot l_pu : Inport  Port=2
  Gain10 : Gain  Gain=1/2
  Moving Average1 : eeGeneralControl/Moving Average  Commented=on  VariantControl=Variant1  LabelModeActiveChoice=Discrete  f=50  x0=0  Ts=-1
      settings: SourceProductBaseCode=PS
  Product : Product
  Product1 : Product
  Second-Order Filter1 : spsSecondOrderFilterLib/Second-Order Filter  FilterType=Bandstop (Notch)  Fo=fb  Zeta=1  Ts=0  Initialize=on  Vac_Init="[0,  0,  60; 0, 0, 60; 0, 0, 60]"  Vdc_Init=[0, 0, 0]  PlotResponse=off  FreqRange=[0, 500, 1]
      settings: SourceProductBaseCode=PS
  Sum3 : Sum  Inputs=+-
  Wdiff : Outport  PortDimensions=3
  wires:
  vctot u_pu/1 -> Product/2, Product/1
  Sum3/1 -> Gain10/1
  vctot l_pu/1 -> Product1/2, Product1/1
  Product/1 -> Sum3/1
  Product1/1 -> Sum3/2
  Second-Order Filter1/1 -> Wdiff/1
  Gain10/1 -> Second-Order Filter1/1

== system GFL_Lib/GFM_VC MMC/Control loops/DC part: stored energy control + differential current control/Wtot computation ==
  vctot u_pu : Inport
  vctot l_pu : Inport  Port=2
  Gain10 : Gain  Gain=1/2
  Moving Average1 : eeGeneralControl/Moving Average  Commented=on  VariantControl=Variant1  LabelModeActiveChoice=Discrete  f=50  x0=1  Ts=-1
      settings: SourceProductBaseCode=PS
  Product : Product
  Product1 : Product
  Second-Order Filter : spsSecondOrderFilterLib/Second-Order Filter  FilterType=Bandstop (Notch)  Fo=2*fb  Zeta=1  Ts=0  Initialize=on  Vac_Init="[0,  0,  60; 0, 0, 60; 0, 0, 60]"  Vdc_Init=[1; 1; 1]  PlotResponse=off  FreqRange=[0, 500, 1]
      settings: SourceProductBaseCode=PS
  Sum3 : Sum
  Wtot : Outport  PortDimensions=3
  wires:
  vctot u_pu/1 -> Product/2, Product/1
  Sum3/1 -> Gain10/1
  vctot l_pu/1 -> Product1/2, Product1/1
  Product/1 -> Sum3/1
  Product1/1 -> Sum3/2
  Second-Order Filter/1 -> Wtot/1
  Gain10/1 -> Second-Order Filter/1

== system GFL_Lib/GFM_VC MMC/Control loops/TVI/dq to phasor ==
  dq_mes : Inport
  Demux : Demux  Outputs=2
      settings: DisplayOption=none
  Sqrt : Sqrt  SaturateOnIntegerOverflow=on
  Sum4 : Sum  Inputs=|++  InputSameDT=on  SaturateOnIntegerOverflow=on  OutDataTypeStr=Inherit: Same as first input
  Vrdird : Product  InputSameDT=on  RndMeth=Zero  SaturateOnIntegerOverflow=on  OutDataTypeStr=Inherit: Same as first input
  Vrqirq : Product  InputSameDT=on  RndMeth=Zero  SaturateOnIntegerOverflow=on  OutDataTypeStr=Inherit: Same as first input
  rms : Outport  VectorParamsAs1DForOutWhenUnconnected=off
  wires:
  Sum4/1 -> Sqrt/1
  Vrqirq/1 -> Sum4/2
  Vrdird/1 -> Sum4/1
  Demux/2 -> Vrqirq/2, Vrqirq/1
  Demux/1 -> Vrdird/2, Vrdird/1
  dq_mes/1 -> Demux/1
  Sqrt/1 -> rms/1

== system GFL_Lib/GFM_VC MMC/Control loops/Transient Damping Resistance/Filter w_LF ==
  e : Inport
  1/T_LP : Gain  Gain=W_TVR  SaturateOnIntegerOverflow=on  OutDataTypeStr=Inherit: Same as input  ParamDataTypeStr=Inherit: Same as input
  Integrator : Integrator  InitialConditionSource=external  InitialCondition=[VSC01_id0*0.04]
  Sum1 : Sum  Inputs=|+-  InputSameDT=on  SaturateOnIntegerOverflow=on  OutDataTypeStr=Inherit: Same as first input
  s : Outport  VectorParamsAs1DForOutWhenUnconnected=off
  wires:
  e/1 -> Sum1/1, Integrator/2
  Integrator/1 -> s/1, Sum1/2
  1/T_LP/1 -> Integrator/1
  Sum1/1 -> 1/T_LP/1

== system GFL_Lib/Mean Model 2-Level L-filter with DC Link/Control loops/Inner Current Control/Current PI control ==
  Is_dq : Inport
  Eg_dqfr : Inport  Port=2
  Is_dq_ref : Inport  Port=3
  w : Inport  Port=4
  Idq_ref_max : Inport  Port=5
  Abs1 : Abs
  Abs2 : Abs
  Constant : Constant  Value=0
  Constant1 : Constant  Value=Vm0_d
  Constant2 : Constant  Value=Vm0_q
  Constant3 : Constant  Value=Filtre_FF
  Constant4 : Constant  Value=Filtre_FF
  Demux{,1..3} (4 alike) : Demux  Outputs=2
  Equal : RelationalOperator  Operator=<=  OutDataTypeStr=boolean  RndMeth=Simplest
  Equal1 : RelationalOperator  Operator=<=  OutDataTypeStr=boolean  RndMeth=Simplest
  Gain : Gain  Gain=m^2
  Gain1 : Gain  Gain=1/m
  LPF1 : Subsystem
  LPF2 : Subsystem
  Mux : Mux  Inputs=[1 1]
  PI_fw_init : Subsystem  AncestorBlock=Control_Lib/PI_fw_init  TreatAsAtomicUnit=on  mask{Kp=Kp_i, Ki=Ki_i}
  PI_fw_init1 : Subsystem  AncestorBlock=Control_Lib/PI_fw_init  TreatAsAtomicUnit=on  mask{Kp=Kp_i, Ki=Ki_i}
  Product : Product  RndMeth=Zero
  Product1 : Product  RndMeth=Zero
  Sum : Sum  Inputs=-+
  Sum1 : Sum
  Switch1 : Switch  Criteria=u2 > Threshold  Threshold=0.5
  Switch2 : Switch  Criteria=u2 > Threshold  Threshold=0.5
  Voltage Compensator 1 : Gain  Gain=Kffi
  Voltage compensator : Gain  Gain=Kffi
  w*Lf_pu : Gain  Gain=Lf_pu
  vm_dq_ref : Outport  InitialOutput=0  VectorParamsAs1DForOutWhenUnconnected=off
  wires:
  Voltage compensator/1 -> Switch2/3, LPF1/1(In1)
  w/1 -> Gain/1
  PI_fw_init1/1(y) -> Mux/2  "vm_q_ref"
  PI_fw_init/1(y) -> Mux/1  "vm_d_ref"
  Product1/1 -> Sum1/1
  Demux/2 -> Abs1/1, PI_fw_init1/1(Ref)
  Mux/1 -> Gain1/1
  Demux1/2 -> PI_fw_init1/2(Meas), Product/1
  w*Lf_pu/1 -> Product/2, Product1/1
  Demux1/1 -> PI_fw_init/2(Meas), Product1/2
  Demux/1 -> PI_fw_init/1(Ref), Abs2/1
  Is_dq_ref/1 -> Demux/1
  Is_dq/1 -> Demux1/1
  Eg_dqfr/1 -> Demux2/1
  Product/1 -> Sum/1
  Sum/1 -> PI_fw_init/3(fw)
  Constant1/1 -> PI_fw_init/4(y0)
  Sum1/1 -> PI_fw_init1/3(fw)
  Constant2/1 -> PI_fw_init1/4(y0)
  Demux2/1 -> Voltage compensator/1
  Demux2/2 -> Voltage Compensator 1/1
  Idq_ref_max/1 -> Demux3/1
  Demux3/1 -> Equal/1
  Demux3/2 -> Equal1/1
  Abs2/1 -> Equal/2
  Abs1/1 -> Equal1/2
  Equal/1 -> PI_fw_init/5(held_integ)
  Equal1/1 -> PI_fw_init1/5(held_integ)
  Gain/1 -> w*Lf_pu/1
  Gain1/1 -> vm_dq_ref/1
  LPF1/1(Out1) -> Switch2/1
  Constant3/1 -> Switch2/2
  Switch2/1 -> Sum/2
  LPF2/1(Out1) -> Switch1/1
  Voltage Compensator 1/1 -> Switch1/3, LPF2/1(In1)
  Constant4/1 -> Switch1/2
  Switch1/1 -> Sum1/2

== system GFL_Lib/Mean Model 2-Level L-filter_old/Control loops/Inner Current Control/Current PI control ==
  Is_dq : Inport
  Eg_dqfr : Inport  Port=2
  Is_dq_ref : Inport  Port=3
  w : Inport  Port=4
  Idq_ref_max : Inport  Port=5
  Abs1 : Abs
  Abs2 : Abs
  Constant : Constant  Value=0
  Constant1 : Constant  Value=Vm0_d
  Constant2 : Constant  Value=Vm0_q
  Constant3 : Constant  Value=Filtre_FF
  Constant4 : Constant  Commented=on  Value=Filtre_FF
  Demux{,1..3} (4 alike) : Demux  Outputs=2
  Equal : RelationalOperator  Operator=<=  OutDataTypeStr=boolean  RndMeth=Simplest
  Equal1 : RelationalOperator  Operator=<=  OutDataTypeStr=boolean  RndMeth=Simplest
  Gain : Gain  Gain=m^2
  Gain1 : Gain  Gain=1/m
  LPF1 : Subsystem
  LPF2 : Subsystem  Commented=on
  Mux : Mux  Inputs=[1 1]
  PI_fw_init : Subsystem  AncestorBlock=Control_Lib/PI_fw_init  TreatAsAtomicUnit=on  mask{Kp=Kp_i, Ki=Ki_i}
  PI_fw_init1 : Subsystem  AncestorBlock=Control_Lib/PI_fw_init  TreatAsAtomicUnit=on  mask{Kp=Kp_i, Ki=Ki_i}
  Product : Product  RndMeth=Zero
  Product1 : Product  RndMeth=Zero
  Sum : Sum  Inputs=-+
  Sum1 : Sum
  Switch1 : Switch  Commented=on  Criteria=u2 > Threshold  Threshold=0.5
  Switch2 : Switch  Criteria=u2 > Threshold  Threshold=0.5
  Voltage Compensator 1 : Gain  Commented=on  Gain=Kffi
  Voltage compensator : Gain  Gain=Kffi
  w*Lf_pu : Gain  Gain=Lf_pu
  vm_dq_ref : Outport  InitialOutput=0  VectorParamsAs1DForOutWhenUnconnected=off
  wires:
  Voltage compensator/1 -> Switch2/3, LPF1/1(In1)
  w/1 -> Gain/1
  Constant2/1 -> Mux/2, PI_fw_init1/4(y0)  "vm_q_ref"
  Constant1/1 -> Mux/1, PI_fw_init/4(y0)  "vm_d_ref"
  Product1/1 -> Sum1/1
  Demux/2 -> Abs1/1, PI_fw_init1/1(Ref)
  Mux/1 -> Gain1/1
  Demux1/2 -> PI_fw_init1/2(Meas), Product/1
  w*Lf_pu/1 -> Product/2, Product1/1
  Demux1/1 -> PI_fw_init/2(Meas), Product1/2
  Demux/1 -> PI_fw_init/1(Ref), Abs2/1
  Is_dq_ref/1 -> Demux/1
  Is_dq/1 -> Demux1/1
  Eg_dqfr/1 -> Demux2/1
  Product/1 -> Sum/1
  Sum/1 -> PI_fw_init/3(fw)
  Sum1/1 -> PI_fw_init1/3(fw)
  Demux2/1 -> Voltage compensator/1
  Demux2/2 -> Voltage Compensator 1/1
  Idq_ref_max/1 -> Demux3/1
  Demux3/1 -> Equal/1
  Demux3/2 -> Equal1/1
  Abs2/1 -> Equal/2
  Abs1/1 -> Equal1/2
  Equal/1 -> PI_fw_init/5(held_integ)
  Equal1/1 -> PI_fw_init1/5(held_integ)
  Gain/1 -> w*Lf_pu/1
  Gain1/1 -> vm_dq_ref/1
  LPF1/1(Out1) -> Switch2/1
  Constant3/1 -> Switch2/2
  Switch2/1 -> Sum/2
  LPF2/1(Out1) -> Switch1/1
  Voltage Compensator 1/1 -> Switch1/3, LPF2/1(In1)
  Constant4/1 -> Switch1/2
  Switch1/1 -> Sum1/2

== system GFL_Lib/Mean Model 2-Level L-filter_sav/Control loops/Inner Current Control/Current PI control ==
  Is_dq : Inport
  Eg_dqfr : Inport  Port=2
  Is_dq_ref : Inport  Port=3
  w : Inport  Port=4
  Constant : Constant
  Constant1 : Constant  Value=Vm0_d
  Constant2 : Constant  Value=Vm0_q
  Constant3 : Constant
  Demux : Demux  Outputs=2
  Demux1 : Demux  Outputs=2
  Demux2 : Demux  Outputs=2
  Mux : Mux  Inputs=[1 1]
  PI_fw_init : Control_Lib/PI_fw_init  Kp=Kp_i  Ki=Ki_i
      settings: SourceProductName=VSC4SPS
  PI_fw_init1 : Control_Lib/PI_fw_init  Kp=Kp_i  Ki=Ki_i
      settings: SourceProductName=VSC4SPS
  Product : Product  RndMeth=Zero
  Product1 : Product  RndMeth=Zero
  Sum : Sum  Inputs=-+
  Sum1 : Sum
  Voltage Compensator 1 : Gain  Gain=Kffi
  Voltage compensator : Gain  Gain=Kffi
  w*Lf_pu : Gain  Gain=Lf_pu
  vm_dq_ref : Outport  InitialOutput=0  VectorParamsAs1DForOutWhenUnconnected=off
  wires:
  Constant3/1 -> PI_fw_init1/5
  Constant2/1 -> PI_fw_init1/4
  Voltage Compensator 1/1 -> Sum1/2
  Sum1/1 -> PI_fw_init1/3
  Constant1/1 -> PI_fw_init/4
  Constant/1 -> PI_fw_init/5
  Sum/1 -> PI_fw_init/3
  Product/1 -> Sum/1
  Eg_dqfr/1 -> Demux2/1
  Demux2/2 -> Voltage Compensator 1/1
  Demux2/1 -> Voltage compensator/1
  Is_dq/1 -> Demux1/1
  Is_dq_ref/1 -> Demux/1
  Demux/1 -> PI_fw_init/1
  Demux1/1 -> Product1/2, PI_fw_init/2
  w*Lf_pu/1 -> Product1/1, Product/2
  Demux1/2 -> Product/1, PI_fw_init1/2
  Mux/1 -> vm_dq_ref/1
  Demux/2 -> PI_fw_init1/1
  Product1/1 -> Sum1/1
  PI_fw_init/1 -> Mux/1  "vm_d_ref"
  PI_fw_init1/1 -> Mux/2  "vm_q_ref"
  w/1 -> w*Lf_pu/1
  Voltage compensator/1 -> Sum/2

== system GFL_Lib/Mean Model 2-Level LCL-filter [under construction]/Control loops/Inner Current Control/Current PI control ==
  Is_dq : Inport
  Eg_dqfr : Inport  Port=2
  Is_dq_ref : Inport  Port=3
  w : Inport  Port=4
  Constant : Constant
  Constant1 : Constant  Value=Vm0_d
  Constant2 : Constant  Value=Vm0_q
  Constant3 : Constant
  Demux : Demux  Outputs=2
  Demux1 : Demux  Outputs=2
  Demux2 : Demux  Outputs=2
  Mux : Mux  Inputs=[1 1]
  PI_fw_init : Control_Lib/PI_fw_init  Kp=Kp_i  Ki=Ki_i
      settings: SourceProductName=VSC4SPS
  PI_fw_init1 : Control_Lib/PI_fw_init  Kp=Kp_i  Ki=Ki_i
      settings: SourceProductName=VSC4SPS
  Product : Product  RndMeth=Zero
  Product1 : Product  RndMeth=Zero
  Sum : Sum  Inputs=-+
  Sum1 : Sum
  Voltage Compensator 1 : Gain  Gain=Kffi
  Voltage compensator : Gain  Gain=Kffi
  w*Lf_pu : Gain  Gain=Lf_pu
  vm_dq_ref : Outport  InitialOutput=0  VectorParamsAs1DForOutWhenUnconnected=off
  wires:
  Constant3/1 -> PI_fw_init1/5
  Constant2/1 -> PI_fw_init1/4
  Voltage Compensator 1/1 -> Sum1/2
  Sum1/1 -> PI_fw_init1/3
  Constant1/1 -> PI_fw_init/4
  Constant/1 -> PI_fw_init/5
  Sum/1 -> PI_fw_init/3
  Product/1 -> Sum/1
  Eg_dqfr/1 -> Demux2/1
  Demux2/2 -> Voltage Compensator 1/1
  Demux2/1 -> Voltage compensator/1
  Is_dq/1 -> Demux1/1
  Is_dq_ref/1 -> Demux/1
  Demux/1 -> PI_fw_init/1
  Demux1/1 -> Product1/2, PI_fw_init/2
  w*Lf_pu/1 -> Product1/1, Product/2
  Demux1/2 -> Product/1, PI_fw_init1/2
  Mux/1 -> vm_dq_ref/1
  Demux/2 -> PI_fw_init1/1
  Product1/1 -> Sum1/1
  PI_fw_init/1 -> Mux/1  "vm_d_ref"
  PI_fw_init1/1 -> Mux/2  "vm_q_ref"
  w/1 -> w*Lf_pu/1
  Voltage compensator/1 -> Sum/2

== system GFL_Lib/Mean Model 2-Level L-filter with DC Link/Control loops/Inner Current Control/Current PI control/LPF1 ==
  In1 : Inport
  Add : Sum  Inputs=+-
  Gain : Gain  Gain=w_ff
  Integrator : Integrator  InitialCondition=V0*cos(Theta0*pi/180)
  Out1 : Outport
  wires:
  In1/1 -> Add/1
  Integrator/1 -> Add/2, Out1/1
  Gain/1 -> Integrator/1
  Add/1 -> Gain/1

== system GFL_Lib/Mean Model 2-Level L-filter with DC Link/Control loops/Inner Current Control/Current PI control/LPF2 ==
  In1 : Inport
  Add : Sum  Inputs=+-
  Gain : Gain  Gain=w_ff
  Integrator : Integrator  InitialCondition=V0*sin(Theta0*pi/180)
  Out1 : Outport
  wires:
  In1/1 -> Add/1
  Integrator/1 -> Add/2, Out1/1
  Gain/1 -> Integrator/1
  Add/1 -> Gain/1

== system GFL_Lib/Mean Model 2-Level L-filter with DC Link/Control loops/Inner Current Control/Current PI control/PI_fw_init ==
  Ref : Inport
  Meas : Inport  Port=2
  fw : Inport  Port=3
  y0 : Inport  Port=4
  held_integ : Inport  Port=5
  Constant : Constant  Value=0
  Constant1 : Constant  Value=0
  Data Type Conversion : DataTypeConversion
  Gain : Gain  Gain=Kp
  Gain1 : Gain  Gain=Ki
  Init_condition : Subsystem
  Integrator : Integrator  InitialConditionSource=external
  Memory : Memory  InitialCondition=1
  Subsystem : Subsystem  Commented=on
  Sum : Sum
  Sum1 : Sum  Inputs=+-
  Sum2 : Sum
  Switch : Switch  Criteria=u2 > Threshold  Threshold=0.5
  y : Outport  VectorParamsAs1DForOutWhenUnconnected=off
  wires:
  Init_condition/1(integ0) -> Integrator/2
  [comp] -> Init_condition/2(comp)
  Ref/1 -> Sum1/1
  Meas/1 -> Sum1/2
  Sum/1 -> Sum2/1, [comp]
  Sum1/1 -> Gain/1, Gain1/1
  Sum2/1 -> y/1
  y0/1 -> Init_condition/1(y0)
  Constant/1 -> Memory/1
  Memory/1 -> Init_condition/Enable
  fw/1 -> Sum/1
  Gain/1 -> Sum/2
  Integrator/1 -> Sum2/2
  Switch/1 -> Integrator/1
  Constant1/1 -> Switch/1
  Gain1/1 -> Switch/3
  held_integ/1 -> Data Type Conversion/1
  Data Type Conversion/1 -> Switch/2

== system GFL_Lib/Mean Model 2-Level L-filter with DC Link/Control loops/Inner Current Control/Current PI control/PI_fw_init1 ==
  Ref : Inport
  Meas : Inport  Port=2
  fw : Inport  Port=3
  y0 : Inport  Port=4
  held_integ : Inport  Port=5
  Constant : Constant  Value=0
  Constant1 : Constant  Value=0
  Data Type Conversion : DataTypeConversion
  Gain : Gain  Gain=Kp
  Gain1 : Gain  Gain=Ki
  Init_condition : Subsystem
  Integrator : Integrator  InitialConditionSource=external
  Memory : Memory  InitialCondition=1
  Subsystem : Subsystem  Commented=on
  Sum : Sum
  Sum1 : Sum  Inputs=+-
  Sum2 : Sum
  Switch : Switch  Criteria=u2 > Threshold  Threshold=0.5
  y : Outport  VectorParamsAs1DForOutWhenUnconnected=off
  wires:
  Init_condition/1(integ0) -> Integrator/2
  [comp] -> Init_condition/2(comp)
  Ref/1 -> Sum1/1
  Meas/1 -> Sum1/2
  Sum/1 -> Sum2/1, [comp]
  Sum1/1 -> Gain/1, Gain1/1
  Sum2/1 -> y/1
  y0/1 -> Init_condition/1(y0)
  Constant/1 -> Memory/1
  Memory/1 -> Init_condition/Enable
  fw/1 -> Sum/1
  Gain/1 -> Sum/2
  Integrator/1 -> Sum2/2
  Switch/1 -> Integrator/1
  Constant1/1 -> Switch/1
  Gain1/1 -> Switch/3
  held_integ/1 -> Data Type Conversion/1
  Data Type Conversion/1 -> Switch/2

== system GFL_Lib/Mean Model 2-Level L-filter_old/Control loops/Inner Current Control/Current PI control/LPF1 ==
  In1 : Inport
  Add : Sum  Inputs=+-
  Gain : Gain  Gain=w_ff
  Integrator : Integrator  InitialCondition=V0*cos(Theta0*pi/180)
  Out1 : Outport
  wires:
  In1/1 -> Add/1
  Integrator/1 -> Add/2, Out1/1
  Gain/1 -> Integrator/1
  Add/1 -> Gain/1

== system GFL_Lib/Mean Model 2-Level L-filter_old/Control loops/Inner Current Control/Current PI control/LPF2 ==
  In1 : Inport
  Add : Sum  Inputs=+-
  Gain : Gain  Gain=w_ff
  Integrator : Integrator  InitialCondition=V0*sin(Theta0*pi/180)
  Out1 : Outport
  wires:
  In1/1 -> Add/1
  Integrator/1 -> Add/2, Out1/1
  Gain/1 -> Integrator/1
  Add/1 -> Gain/1

== system GFL_Lib/Mean Model 2-Level L-filter_old/Control loops/Inner Current Control/Current PI control/PI_fw_init ==
  Ref : Inport
  Meas : Inport  Port=2
  fw : Inport  Port=3
  y0 : Inport  Port=4
  held_integ : Inport  Port=5
  Constant : Constant  Value=0
  Constant1 : Constant  Value=0
  Data Type Conversion : DataTypeConversion
  Gain : Gain  Gain=Kp
  Gain1 : Gain  Gain=Ki
  Init_condition : Subsystem
  Integrator : Integrator  InitialConditionSource=external
  Memory : Memory  InitialCondition=1
  Subsystem : Subsystem  Commented=on
  Sum : Sum
  Sum1 : Sum  Inputs=+-
  Sum2 : Sum
  Switch : Switch  Criteria=u2 > Threshold  Threshold=0.5
  y : Outport  VectorParamsAs1DForOutWhenUnconnected=off
  wires:
  Init_condition/1(integ0) -> Integrator/2
  [comp] -> Init_condition/2(comp)
  Ref/1 -> Sum1/1
  Meas/1 -> Sum1/2
  Sum/1 -> Sum2/1, [comp]
  Sum1/1 -> Gain/1, Gain1/1
  Sum2/1 -> y/1
  y0/1 -> Init_condition/1(y0)
  Constant/1 -> Memory/1
  Memory/1 -> Init_condition/Enable
  fw/1 -> Sum/1
  Gain/1 -> Sum/2
  Integrator/1 -> Sum2/2
  Switch/1 -> Integrator/1
  Constant1/1 -> Switch/1
  Gain1/1 -> Switch/3
  held_integ/1 -> Data Type Conversion/1
  Data Type Conversion/1 -> Switch/2

== system GFL_Lib/Mean Model 2-Level L-filter_old/Control loops/Inner Current Control/Current PI control/PI_fw_init1 ==
  Ref : Inport
  Meas : Inport  Port=2
  fw : Inport  Port=3
  y0 : Inport  Port=4
  held_integ : Inport  Port=5
  Constant : Constant  Value=0
  Constant1 : Constant  Value=0
  Data Type Conversion : DataTypeConversion
  Gain : Gain  Gain=Kp
  Gain1 : Gain  Gain=Ki
  Init_condition : Subsystem
  Integrator : Integrator  InitialConditionSource=external
  Memory : Memory  InitialCondition=1
  Subsystem : Subsystem  Commented=on
  Sum : Sum
  Sum1 : Sum  Inputs=+-
  Sum2 : Sum
  Switch : Switch  Criteria=u2 > Threshold  Threshold=0.5
  y : Outport  VectorParamsAs1DForOutWhenUnconnected=off
  wires:
  Init_condition/1(integ0) -> Integrator/2
  [comp] -> Init_condition/2(comp)
  Ref/1 -> Sum1/1
  Meas/1 -> Sum1/2
  Sum/1 -> Sum2/1, [comp]
  Sum1/1 -> Gain/1, Gain1/1
  Sum2/1 -> y/1
  y0/1 -> Init_condition/1(y0)
  Constant/1 -> Memory/1
  Memory/1 -> Init_condition/Enable
  fw/1 -> Sum/1
  Gain/1 -> Sum/2
  Integrator/1 -> Sum2/2
  Switch/1 -> Integrator/1
  Constant1/1 -> Switch/1
  Gain1/1 -> Switch/3
  held_integ/1 -> Data Type Conversion/1
  Data Type Conversion/1 -> Switch/2

== system GFL_Lib/Mean Model 2-Level L-filter with DC Link/Control loops/Inner Current Control/Current PI control/PI_fw_init/Init_condition ==
  y0 : Inport
  comp : Inport  Port=2
  Enable : EnablePort
  Sum : Sum  Inputs=-+
  integ0 : Outport  VectorParamsAs1DForOutWhenUnconnected=off
  wires:
  Sum/1 -> integ0/1
  y0/1 -> Sum/2
  comp/1 -> Sum/1

== system GFL_Lib/Mean Model 2-Level L-filter with DC Link/Control loops/Inner Current Control/Current PI control/PI_fw_init/Subsystem ==
  e : Inport
  x0 : Inport  Port=2
  Enable : EnablePort
  Integrator : Integrator  InitialConditionSource=external
  y : Outport  VectorParamsAs1DForOutWhenUnconnected=off
  wires:
  x0/1 -> Integrator/2
  Integrator/1 -> y/1
  e/1 -> Integrator/1

== system GFL_Lib/Mean Model 2-Level L-filter with DC Link/Control loops/Inner Current Control/Current PI control/PI_fw_init1/Init_condition ==
  y0 : Inport
  comp : Inport  Port=2
  Enable : EnablePort
  Sum : Sum  Inputs=-+
  integ0 : Outport  VectorParamsAs1DForOutWhenUnconnected=off
  wires:
  Sum/1 -> integ0/1
  y0/1 -> Sum/2
  comp/1 -> Sum/1
